simulink model "Main"  (R2024a)
settings: Solver=FixedStepAuto  StartTime=0.0  StopTime=150.17  FixedStep=0.002  RelTol=1e-3
undefined symbols (not defined in the file): Estimatex, Estimatey, Estimatez
libraries: dspindex x10, simulink_extras x3, uavsim3dlib x3, sim3dlib x1
settings Model: SnapshotInterval=1  Creator=Guy  LastModifiedBy=dylanfanner
settings OptimizationCC: ReuseModelBlockBuffer=off
settings ModelReferenceCC: EnableRefExpFcnMdlSchedulingChecks=on
settings RTWCC: GPUComputeCapability=3.5

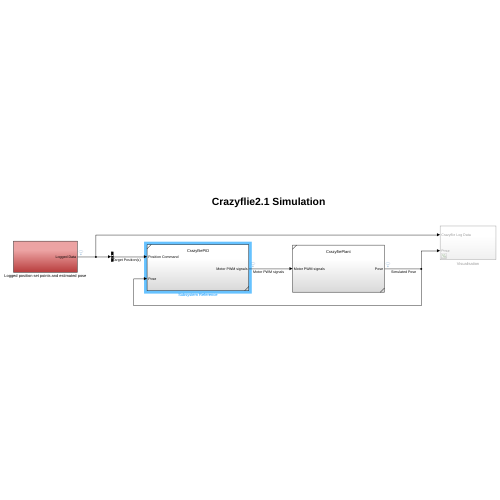
[thumbnail: Simulink's stored preview of the top-level diagram]
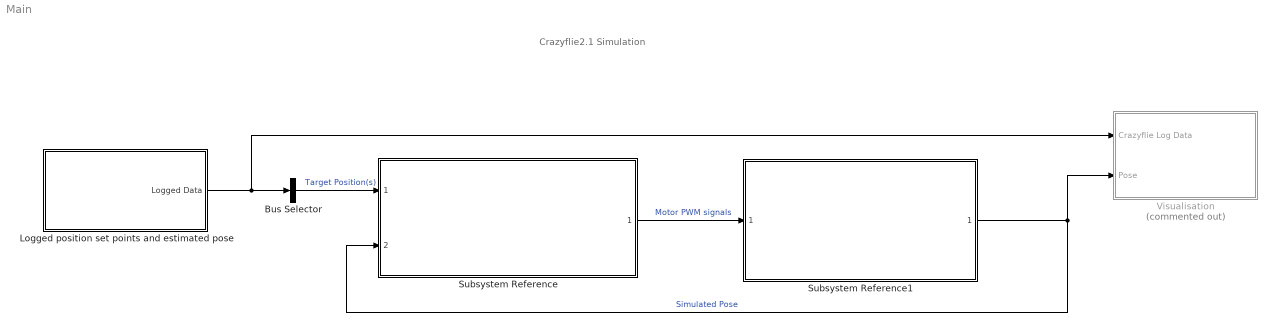
== system Main ==
  note: Crazyflie2.1 Simulation
  Bus Selector : BusSelector  OutputSignals=x,y,z,yaw  OutputAsBus=on
  Logged position set points and estimated pose : Subsystem  Tag=Signal Editor
  Subsystem Reference : Subsystem  ReferencedSubsystem=CrazyfliePID
  Subsystem Reference1 : Subsystem  ReferencedSubsystem=CrazyfliePlant
  Visualisation : Subsystem  Commented=on
  wires:
  Bus Selector/1 -> Subsystem Reference/1  "Target Position(s)"
  Subsystem Reference1/1 -> Visualisation/2(Pose), Subsystem Reference/2  "Simulated Pose"
  Subsystem Reference/1 -> Subsystem Reference1/1  "Motor PWM signals"
  Logged position set points and estimated pose/1(Logged Data) -> Visualisation/1(Crazyflie Log Data), Bus Selector/1

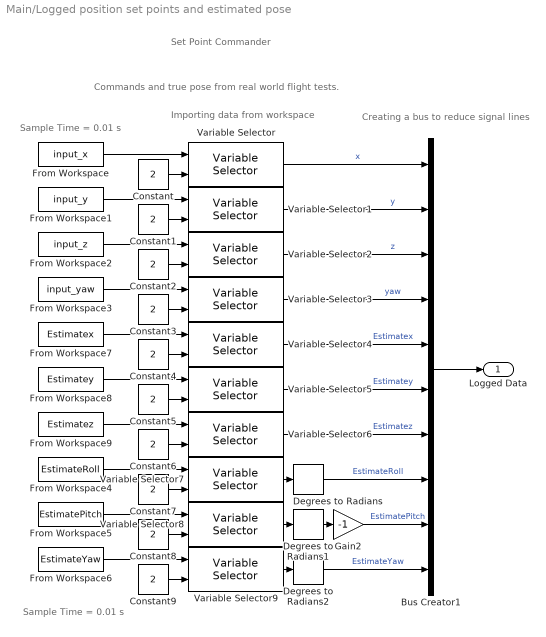
== system Main/Logged position set points and estimated pose ==
  note: Creating a bus to reduce signal lines
  note: Set Point Commander
  note: Importing data from workspace
  note: Commands and true pose from real world flight tests.
  note: Sample Time = 0.01 s
  note: Sample Time = 0.01 s
  Bus Creator1 : BusCreator  Inputs=10
  Constant{,1..9} (10 alike) : Constant  Value=2
  Degrees to Radians : simulink_extras/Transformations/Degrees to Radians
  Degrees to Radians1 : simulink_extras/Transformations/Degrees to Radians
  Degrees to Radians2 : simulink_extras/Transformations/Degrees to Radians
  From Workspace : FromWorkspace  VariableName=input_x  SampleTime=0.01  OutputAfterFinalValue=Holding final value
  From Workspace1 : FromWorkspace  VariableName=input_y  SampleTime=0.01  OutputAfterFinalValue=Setting to zero
  From Workspace2 : FromWorkspace  VariableName=input_z  SampleTime=0.01  OutputAfterFinalValue=Setting to zero
  From Workspace3 : FromWorkspace  VariableName=input_yaw  SampleTime=0.01  OutputAfterFinalValue=Setting to zero
  From Workspace4 : FromWorkspace  VariableName=EstimateRoll  SampleTime=0.002  OutputAfterFinalValue=Setting to zero
  From Workspace5 : FromWorkspace  VariableName=EstimatePitch  SampleTime=0.002  OutputAfterFinalValue=Setting to zero
  From Workspace6 : FromWorkspace  VariableName=EstimateYaw  SampleTime=0.002  OutputAfterFinalValue=Setting to zero
  From Workspace7 : FromWorkspace  VariableName=Estimatex  SampleTime=0.002  OutputAfterFinalValue=Setting to zero
  From Workspace8 : FromWorkspace  VariableName=Estimatey  SampleTime=0.002  OutputAfterFinalValue=Setting to zero
  From Workspace9 : FromWorkspace  VariableName=Estimatez  SampleTime=0.002  OutputAfterFinalValue=Setting to zero
  Gain2 : Gain  Gain=-1
  Variable Selector{,1..9} (10 alike) : dspindex/Variable Selector  NumInputs=1  rowsOrCols=Columns  IdxMode=Variable  Elements=[1 3]  ZerOneIdxMode=One-based  errmode=Clip Index  FillMode=off  FillValues=0
  Logged Data : Outport
  wires:
  From Workspace/1 -> Variable Selector/1
  Bus Creator1/1 -> Logged Data/1
  From Workspace1/1 -> Variable Selector1/1
  From Workspace2/1 -> Variable Selector2/1
  From Workspace3/1 -> Variable Selector3/1
  Variable Selector6/1 -> Bus Creator1/7  "Estimatez"
  Variable Selector5/1 -> Bus Creator1/6  "Estimatey"
  Variable Selector4/1 -> Bus Creator1/5  "Estimatex"
  Variable Selector3/1 -> Bus Creator1/4  "yaw"
  Variable Selector2/1 -> Bus Creator1/3  "z"
  Variable Selector1/1 -> Bus Creator1/2  "y"
  Variable Selector/1 -> Bus Creator1/1  "x"
  Constant1/1 -> Variable Selector1/2
  Constant/1 -> Variable Selector/2
  Constant2/1 -> Variable Selector2/2
  Constant3/1 -> Variable Selector3/2
  Constant4/1 -> Variable Selector4/2
  Constant5/1 -> Variable Selector5/2
  Constant6/1 -> Variable Selector6/2
  Constant7/1 -> Variable Selector7/2
  Variable Selector7/1 -> Degrees to Radians/1
  Constant8/1 -> Variable Selector8/2
  Constant9/1 -> Variable Selector9/2
  Variable Selector9/1 -> Degrees to Radians2/1
  From Workspace7/1 -> Variable Selector4/1
  From Workspace8/1 -> Variable Selector5/1
  From Workspace9/1 -> Variable Selector6/1
  From Workspace4/1 -> Variable Selector7/1
  From Workspace5/1 -> Variable Selector8/1
  From Workspace6/1 -> Variable Selector9/1
  Gain2/1 -> Bus Creator1/9  "EstimatePitch"
  Degrees to Radians/1 -> Bus Creator1/8  "EstimateRoll"
  Variable Selector8/1 -> Degrees to Radians1/1
  Degrees to Radians1/1 -> Gain2/1
  Degrees to Radians2/1 -> Bus Creator1/10  "EstimateYaw"

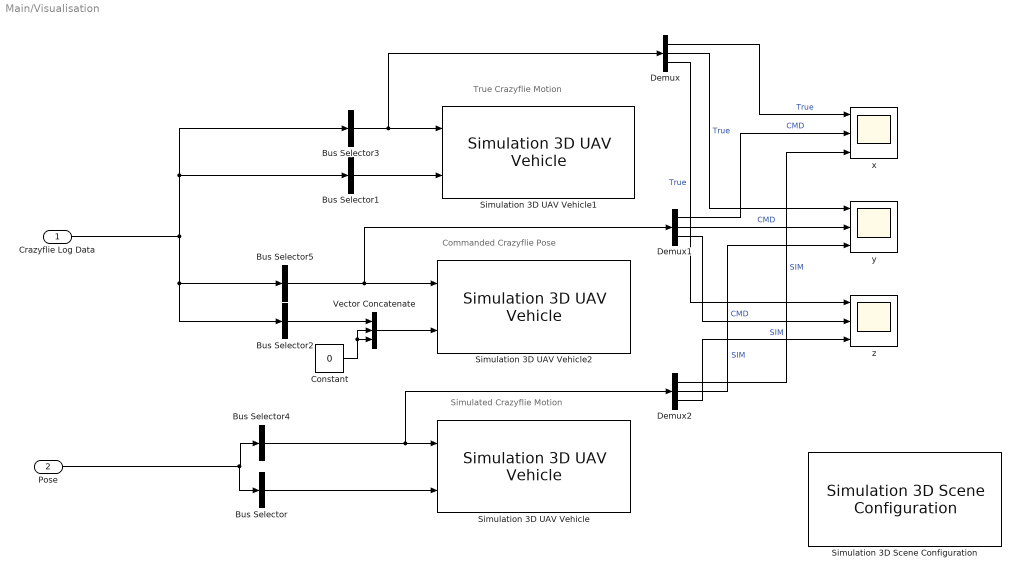
== system Main/Visualisation ==
  note: True Crazyflie Motion
  note: Commanded Crazyflie Pose
  note: Simulated Crazyflie Motion
  Crazyflie Log Data : Inport
  Pose : Inport  Port=2
  Bus Selector : BusSelector  OutputSignals=Attitude State.attitude.ψ,Attitude State.attitude.θ,Attitude State.attitude.Φ  OutputAsBus=on
  Bus Selector1 : BusSelector  OutputSignals=EstimateYaw,EstimatePitch,EstimateRoll  OutputAsBus=on
  Bus Selector2 : BusSelector  OutputSignals=yaw  OutputAsBus=on
  Bus Selector3 : BusSelector  OutputSignals=Estimatex,Estimatey,Estimatez  OutputAsBus=on
  Bus Selector4 : BusSelector  OutputSignals=Position State.position.x,Position State.position.y,Position State.position.z  OutputAsBus=on
  Bus Selector5 : BusSelector  OutputSignals=x,y,z  OutputAsBus=on
  Constant : Constant  Value=0
  Demux : Demux  Outputs=3
  Demux1 : Demux  Outputs=3
  Demux2 : Demux  Outputs=3
  Simulation 3D Scene Configuration : sim3dlib/Simulation 3D Scene Configuration  Priority=0  ProjectFormat=Default Scenes  SceneDesc=US city block  ProjectName=C:\Program Files\MATLAB\R2024a\toolbox\shared\sim3d_projects\automotive_project_windows\UE\WindowsNoEditor\VehicleSimulation.exe  ScenePath=/Game/Maps/USCityBlock  EnableOpenDRIVE=off  vehTagList={'Custom';'Scene Origin';'SimulinkVehicle1';'SimulinkVehicle2';'SimulinkVehicle3'}  vehTag=Custom  FreeCameraInitialTranslation=[-2, 1.5, 1.5]  FreeCameraDefaultInitialTranslation=[-6, 0, 2]  FreeCameraInitialRotation=[0, -10, -30]  FreeCameraDefaultInitialRotation=[0, -15, 0]  OpVisEn=off  Ts=0.03  EnableWindow=on  EnableRemoteAccess=off  EnableWeather=off  SunAzimuth=90  SunAltitude=40.0  EnableGeospatialSun=off  Latitude=0  Longitude=0  Date=2023-01-01  Time=10:30:00  GeoTimeZone=-5.0  SunDaylightSaving=off  wind=1  clouds=10  EnableVolumetricClouds=off  CloudCoverage=0  CloudAltitude=6  fog=0  rain=0  RaindropsEffect=off  SnowDensity=0  EnableGeospatial=off  UseTrueOrigin=off  OriginHeight=200  OriginLatitude=40.744652  OriginLongitude=-73.988864  MapStyle=Aerial  AdditionalAssetIDs=[]  UseAdvancedSunSky=off  SolarTime=11  TimeZone=-5  Day=21  Month=9  Year=2022  UseDaylightSavingTime=on  DSTStartDay=10  DSTStartMonth=3  DSTEndDay=3  DSTEndMonth=11  DSTSwitchHour=2  sensorTag=MainCamera1  sensorId=1  sensorName=MainCamera1  mountLoc=Origin  offsetFlag=off  tmountOffset=[0, 0, 0]  rmountOffset=[0, 0, 0]  HorizontalResolution=1280  VerticalResolution=720  HorizontalFOV=60  mountPoint=[0 0 0]  mountOrientation=[0 0 0]  aMode=4  ID=1  GeoTrigger=Inactive
      settings: LibrarySourceBlock=uavsim3dlib/Simulation 3D Scene Configuration
  Simulation 3D UAV Vehicle : uavsim3dlib/Simulation 3D UAV Vehicle  Priority=-1  Mesh=Quadrotor  MeshPath=/MathWorksUAVContent/UAVs/HexaRotorUAV/HexaRotor.HexaRotor  Color=Black  ActorName=SimulinkVehicle1  UseGlobalFrame=off  InitialTranslation=[0 0 0]  InitialRotation=[0 0 0]  InitialTranslationGlobal=[0 0 0]  InitialGeoOrigin=[0 0 0]  InitialRotationGlobal=[0 0 0]  SampleTime=-1  ActorType=SimulinkVehicle  ID=1  aMode=4  ActorTag=SimulinkVehicle1
  Simulation 3D UAV Vehicle1 : uavsim3dlib/Simulation 3D UAV Vehicle  Priority=-1  Mesh=Quadrotor  MeshPath=/MathWorksUAVContent/UAVs/HexaRotorUAV/HexaRotor.HexaRotor  Color=Green  ActorName=SimulinkVehicle2  UseGlobalFrame=off  InitialTranslation=[Estimatex(1,2) Estimatey(1,2) Estimatez(1,2)]  InitialRotation=[0 0 0]  InitialTranslationGlobal=[0 0 0]  InitialGeoOrigin=[0 0 0]  InitialRotationGlobal=[0 0 0]  SampleTime=-1  ActorType=SimulinkVehicle  ID=2  aMode=4  ActorTag=SimulinkVehicle2
  Simulation 3D UAV Vehicle2 : uavsim3dlib/Simulation 3D UAV Vehicle  Priority=-1  Mesh=Quadrotor  MeshPath=/MathWorksUAVContent/UAVs/HexaRotorUAV/HexaRotor.HexaRotor  Color=Black  ActorName=SimulinkVehicle3  UseGlobalFrame=off  InitialTranslation=[0 0 0]  InitialRotation=[0 0 0]  InitialTranslationGlobal=[0 0 0]  InitialGeoOrigin=[0 0 0]  InitialRotationGlobal=[0 0 0]  SampleTime=-1  ActorType=SimulinkVehicle  ID=3  aMode=4  ActorTag=SimulinkVehicle3
  Vector Concatenate : Concatenate  NumInputs=3
  x : Scope  NumInputPorts=3
  y : Scope  NumInputPorts=3
  z : Scope  NumInputPorts=3
  wires:
  Crazyflie Log Data/1 -> Bus Selector5/1, Bus Selector2/1, Bus Selector3/1, Bus Selector1/1
  Bus Selector1/1 -> Simulation 3D UAV Vehicle1/2
  Bus Selector/1 -> Simulation 3D UAV Vehicle/2
  Bus Selector3/1 -> Demux/1, Simulation 3D UAV Vehicle1/1
  Bus Selector5/1 -> Demux1/1, Simulation 3D UAV Vehicle2/1
  Pose/1 -> Bus Selector/1, Bus Selector4/1
  Bus Selector4/1 -> Demux2/1, Simulation 3D UAV Vehicle/1
  Bus Selector2/1 -> Vector Concatenate/1
  Constant/1 -> Vector Concatenate/2, Vector Concatenate/3
  Vector Concatenate/1 -> Simulation 3D UAV Vehicle2/2
  Demux/1 -> x/1  "True"
  Demux1/1 -> x/2  "CMD"
  Demux2/1 -> x/3  "SIM"
  Demux/2 -> y/1  "True"
  Demux1/2 -> y/2  "CMD"
  Demux2/2 -> y/3  "SIM"
  Demux1/3 -> z/2  "CMD"
  Demux/3 -> z/1  "True"
  Demux2/3 -> z/3  "SIM"
